simulink model "Reusable_Model"  (R2021b)
settings: Solver=VariableStepAuto  StartTime=0.0  StopTime=10.0  RelTol=1e-3
settings Model: Creator=amr_y  LastModifiedBy=amr_y

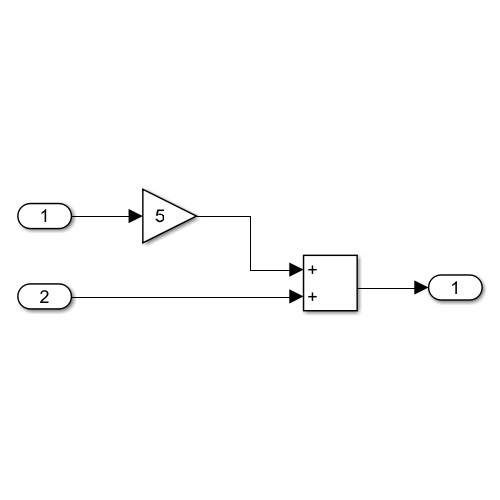
[thumbnail: Simulink's stored preview of the top-level diagram]
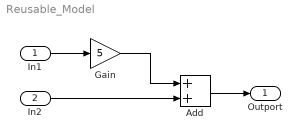
== system Reusable_Model ==
  In1 : Inport
  In2 : Inport  Port=2
  Add : Sum
  Gain : Gain  Gain=5
  Outport : Outport
  wires:
  In2/1 -> Add/2
  Gain/1 -> Add/1
  In1/1 -> Gain/1
  Add/1 -> Outport/1
